simulink model "Circuito"  (R2014a)
settings: Solver=ode45  StartTime=0.0  StopTime=periodo  RelTol=1e-3
PreLoadFcn:
  | variables
InitFcn:
  | eval('variables');
  | variables
StartFcn:
  | variables
undefined symbols (not defined in the file): C, E, frecuencia, L, R, Rc, Rf, Rl, Rml
libraries: fl_lib x63, nesl_utility x4
settings Model: Creator=jhoan  LastModifiedBy=jhoan

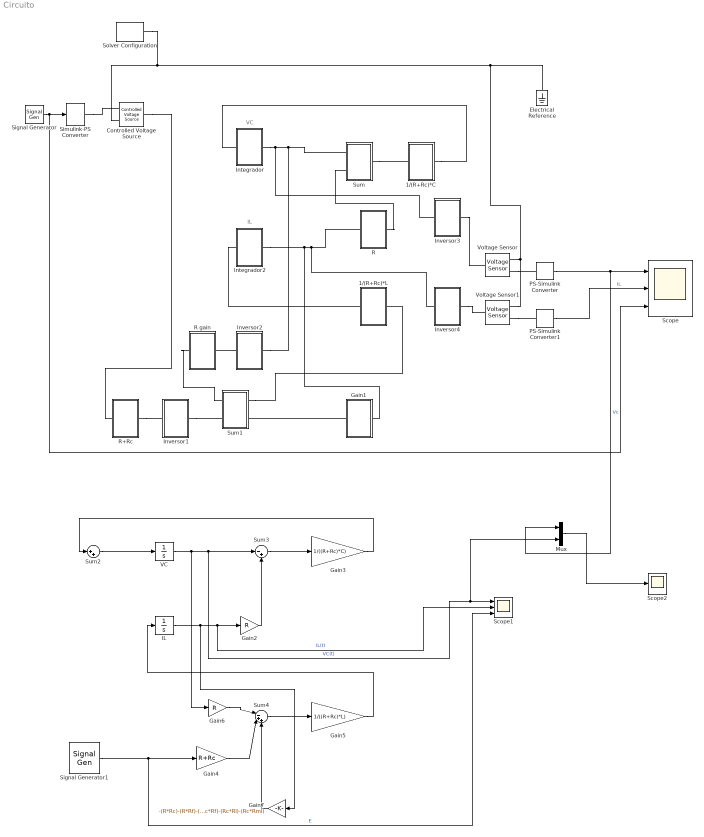
== system Circuito ==
  note: IL
  note: VC
  1/(R+Rc)*C : Subsystem
  1/(R+Rc)*L : Subsystem
  Controlled Voltage Source : fl_lib/Electrical/Electrical Sources/Controlled Voltage Source
  Electrical Reference : fl_lib/Electrical/Electrical Elements/Electrical Reference
  Gain1 : Subsystem
  Gain2 : Gain  Gain=R
  Gain3 : Gain  Gain=1/((R+Rc)*C)
  Gain4 : Gain  Gain=R+Rc
  Gain5 : Gain  Gain=1/((R+Rc)*L)
  Gain6 : Gain  Gain=R
  Gain7 : Gain  Gain=-(R*Rc)-(R*Rf)-(R*Rl)-(R*Rml)-(Rc*Rf)-(Rc*Rl)-(Rc*Rml)
  IL : Integrator
  Integrador : Subsystem
  Integrador2 : Subsystem
  Inversor1 : Subsystem
  Inversor2 : Subsystem
  Inversor3 : Subsystem
  Inversor4 : Subsystem
  Mux : Mux  Inputs=2
  PS-Simulink Converter : nesl_utility/PS-Simulink Converter  PhysicalDomain=network_engine_domain  SubClassName=ps_output  LeftPortType=input  RightPortType=output  PseudoPeriodic=off  Frequencies=[]  Unit=1  AffineConversion=off
  PS-Simulink Converter1 : nesl_utility/PS-Simulink Converter  PhysicalDomain=network_engine_domain  SubClassName=ps_output  LeftPortType=input  RightPortType=output  PseudoPeriodic=off  Frequencies=[]  Unit=1  AffineConversion=off
  R : Subsystem
  R gain : Subsystem
  R+Rc : Subsystem
  Scope : Scope  NumInputPorts=3
      settings: YMin=-5~-5~-5  YMax=5~5~5
  Scope1 : Scope  NumInputPorts=3
      settings: YMin=-5~-5~-5  YMax=5~5~5  SaveName=subSimulink
  Scope2 : Scope
      settings: SaveName=subSimulink1
  Signal Generator : SignalGenerator  WaveForm=square  Amplitude=E  Frequency=frecuencia
  Signal Generator1 : SignalGenerator  WaveForm=square  Amplitude=E  Frequency=frecuencia
  Simulink-PS Converter : nesl_utility/Simulink-PS Converter  PhysicalDomain=network_engine_domain  SubClassName=ps_input  LeftPortType=input  RightPortType=output  PseudoPeriodic=off  Frequencies=[]  NoiseDistribution=none  NoiseParameters=[]  Unit=1  AffineConversion=off  InputFiltering=off  SimscapeFilterOrder=1  InputFilterTimeConstant=0.001  UdotUserProvided=1
  Solver Configuration : nesl_utility/Solver Configuration  PhysicalDomain=network_engine_domain  SubClassName=solver  LeftPortType=input  RightPortType=generic  Accelerate=off  Tones=[]  Harmonics=[]  SimulateNoise=off  Profile=off  UseLocalSampling=off  EnableSwitchedLinearOptims=on  FrequencyDomain=off  UseCCode=off  RelTol=0.001  AbsTol=1e-06  MinStep=1e-09  ToWorkspace=off  DoDC=off  ResidualTolerance=1e-09  UseLocalSolver=off  LocalSolverChoice=NE_BACKWARD_EULER_ADVANCER  LocalSolverSampleTime=0.001  DoFixedCost=off  MaxNonlinIter=3  MaxModeIter=2  LinearAlgebra=Sparse  DelaysMemoryBudget=1024  AutomaticFiltering=on  FilteringTimeConstant=0.001
  Sum : Subsystem
  Sum1 : Subsystem
  Sum2 : Sum  Inputs=|++
  Sum3 : Sum  Inputs=|-+
  Sum4 : Sum  Inputs=|-++
  VC : Integrator
  Voltage Sensor : fl_lib/Electrical/Electrical Sensors/Voltage Sensor
  Voltage Sensor1 : fl_lib/Electrical/Electrical Sensors/Voltage Sensor
  wires:
  PS-Simulink Converter/1 -> Mux/1, Scope/1  "Vc"
  PS-Simulink Converter1/1 -> Scope/2  "IL"
  Signal Generator/1 -> Scope/3, Simulink-PS Converter/1
  Sum2/1 -> VC/1
  IL/1 -> Gain7/1, Scope1/2, Gain2/1  "IL(t)"
  VC/1 -> Gain6/1, Mux/2, Scope1/1, Sum3/1  "VC(t)"
  Gain2/1 -> Sum3/2
  Sum3/1 -> Gain3/1
  Gain3/1 -> Sum2/1
  Signal Generator1/1 -> Scope1/3, Gain4/1  "E"
  Gain4/1 -> Sum4/2
  Sum4/1 -> Gain5/1
  Gain6/1 -> Sum4/1
  Gain5/1 -> IL/1
  Gain7/1 -> Sum4/3
  Mux/1 -> Scope2/1
  connections:
  Solver Configuration/RConn1 -- Controlled Voltage Source/RConn2 -- Electrical Reference/LConn1 -- Voltage Sensor1/RConn2 -- Voltage Sensor/RConn2
  Integrador/RConn1 -- Inversor3/LConn1 -- Inversor2/LConn1 -- Sum/LConn1
  Integrador2/RConn1 -- Gain1/LConn1 -- Inversor4/LConn1 -- R/LConn1
  R/RConn1 -- Sum/LConn2
  Sum/RConn1 -- 1/(R+Rc)*C/LConn1
  1/(R+Rc)*C/RConn1 -- Integrador/LConn1
  Voltage Sensor/RConn1 -- PS-Simulink Converter/LConn1
  Simulink-PS Converter/RConn1 -- Controlled Voltage Source/RConn1
  Controlled Voltage Source/LConn1 -- R+Rc/LConn1
  Inversor2/RConn1 -- R gain/LConn1
  R gain/RConn1 -- Sum1/LConn1
  Sum1/RConn1 -- 1/(R+Rc)*L/LConn1
  1/(R+Rc)*L/RConn1 -- Integrador2/LConn1
  Voltage Sensor1/RConn1 -- PS-Simulink Converter1/LConn1
  R+Rc/RConn1 -- Inversor1/LConn1
  Inversor1/RConn1 -- Sum1/LConn2
  Gain1/RConn1 -- Sum1/RConn2
  Inversor3/RConn1 -- Voltage Sensor/LConn1
  Inversor4/RConn1 -- Voltage Sensor1/LConn1

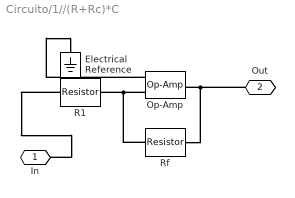
== system Circuito/1//(R+Rc)*C ==
  Electrical Reference : fl_lib/Electrical/Electrical Elements/Electrical Reference
  Op-Amp : fl_lib/Electrical/Electrical Elements/Op-Amp  outI_specify=off  outI_priority=High  outI=0 A
  R1 : fl_lib/Electrical/Electrical Elements/Resistor  R=(R+Rc)*C Ohm  i_specify=off  i_priority=High  i=0 A  v_specify=off  v_priority=High  v=0 V
  Rf : fl_lib/Electrical/Electrical Elements/Resistor  R=1 Ohm  i_specify=off  i_priority=High  i=0 A  v_specify=off  v_priority=High  v=0 V
  In : PMIOPort  Port=1  Side=Left
  Out : PMIOPort  Port=2  Side=Right
  connections:
  R1/LConn1 -- In/RConn1
  Out/RConn1 -- Rf/RConn1 -- Op-Amp/RConn1
  Op-Amp/LConn1 -- Electrical Reference/LConn1
  Op-Amp/LConn2 -- Rf/LConn1 -- R1/RConn1

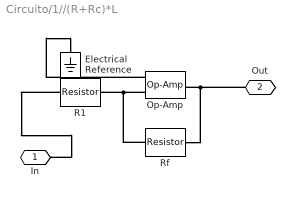
== system Circuito/1//(R+Rc)*L ==
  Electrical Reference : fl_lib/Electrical/Electrical Elements/Electrical Reference
  Op-Amp : fl_lib/Electrical/Electrical Elements/Op-Amp  outI_specify=off  outI_priority=High  outI=0 A
  R1 : fl_lib/Electrical/Electrical Elements/Resistor  R=(R+Rc)*L Ohm  i_specify=off  i_priority=High  i=0 A  v_specify=off  v_priority=High  v=0 V
  Rf : fl_lib/Electrical/Electrical Elements/Resistor  R=1 Ohm  i_specify=off  i_priority=High  i=0 A  v_specify=off  v_priority=High  v=0 V
  In : PMIOPort  Port=1  Side=Left
  Out : PMIOPort  Port=2  Side=Right
  connections:
  R1/LConn1 -- In/RConn1
  Out/RConn1 -- Rf/RConn1 -- Op-Amp/RConn1
  Op-Amp/LConn1 -- Electrical Reference/LConn1
  Op-Amp/LConn2 -- Rf/LConn1 -- R1/RConn1

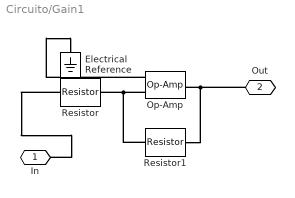
== system Circuito/Gain1 ==
  Electrical Reference : fl_lib/Electrical/Electrical Elements/Electrical Reference
  Op-Amp : fl_lib/Electrical/Electrical Elements/Op-Amp  outI_specify=off  outI_priority=High  outI=0 A
  Resistor : fl_lib/Electrical/Electrical Elements/Resistor  R=1 Ohm  i_specify=off  i_priority=High  i=0 A  v_specify=off  v_priority=High  v=0 V
  Resistor1 : fl_lib/Electrical/Electrical Elements/Resistor  R=(R*Rc)+(R*Rf)+(R*Rl)+(R*Rml)+(Rc*Rf)+(Rc*Rl)+(Rc*Rml) Ohm  i_specify=off  i_priority=High  i=0 A  v_specify=off  v_priority=High  v=0 V
  In : PMIOPort  Port=1  Side=Left
  Out : PMIOPort  Port=2  Side=Right
  connections:
  Resistor/LConn1 -- In/RConn1
  Out/RConn1 -- Resistor1/RConn1 -- Op-Amp/RConn1
  Op-Amp/LConn1 -- Electrical Reference/LConn1
  Op-Amp/LConn2 -- Resistor1/LConn1 -- Resistor/RConn1

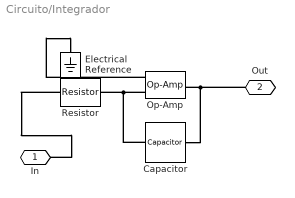
== system Circuito/Integrador ==
  Capacitor : fl_lib/Electrical/Electrical Elements/Capacitor  c=1e-6 F  r=1e-6 Ohm  g=0 1/Ohm  i_specify=off  i_priority=High  i=0 A  v_specify=off  v_priority=High  v=0 V  vc_specify=off  vc_priority=High  vc=0 V
  Electrical Reference : fl_lib/Electrical/Electrical Elements/Electrical Reference
  Op-Amp : fl_lib/Electrical/Electrical Elements/Op-Amp  outI_specify=off  outI_priority=High  outI=0 A
  Resistor : fl_lib/Electrical/Electrical Elements/Resistor  R=1 MOhm  i_specify=off  i_priority=High  i=0 A  v_specify=off  v_priority=High  v=0 V
  In : PMIOPort  Port=1  Side=Left
  Out : PMIOPort  Port=2  Side=Right
  connections:
  Resistor/LConn1 -- In/RConn1
  Capacitor/RConn1 -- Out/RConn1 -- Op-Amp/RConn1
  Op-Amp/LConn1 -- Electrical Reference/LConn1
  Op-Amp/LConn2 -- Capacitor/LConn1 -- Resistor/RConn1

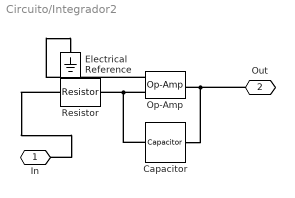
== system Circuito/Integrador2 ==
  Capacitor : fl_lib/Electrical/Electrical Elements/Capacitor  c=1e-6 F  r=1e-6 Ohm  g=0 1/Ohm  i_specify=off  i_priority=High  i=0 A  v_specify=off  v_priority=High  v=0 V  vc_specify=off  vc_priority=High  vc=0 V
  Electrical Reference : fl_lib/Electrical/Electrical Elements/Electrical Reference
  Op-Amp : fl_lib/Electrical/Electrical Elements/Op-Amp  outI_specify=off  outI_priority=High  outI=0 A
  Resistor : fl_lib/Electrical/Electrical Elements/Resistor  R=1 MOhm  i_specify=off  i_priority=High  i=0 A  v_specify=off  v_priority=High  v=0 V
  In : PMIOPort  Port=1  Side=Left
  Out : PMIOPort  Port=2  Side=Right
  connections:
  Resistor/LConn1 -- In/RConn1
  Capacitor/RConn1 -- Out/RConn1 -- Op-Amp/RConn1
  Op-Amp/LConn1 -- Electrical Reference/LConn1
  Op-Amp/LConn2 -- Capacitor/LConn1 -- Resistor/RConn1

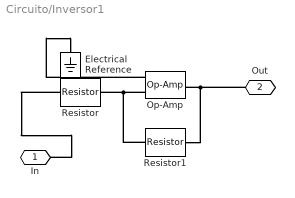
== system Circuito/Inversor1 ==
  Electrical Reference : fl_lib/Electrical/Electrical Elements/Electrical Reference
  Op-Amp : fl_lib/Electrical/Electrical Elements/Op-Amp  outI_specify=off  outI_priority=High  outI=0 A
  Resistor : fl_lib/Electrical/Electrical Elements/Resistor  R=1 kOhm  i_specify=off  i_priority=High  i=0 A  v_specify=off  v_priority=High  v=0 V
  Resistor1 : fl_lib/Electrical/Electrical Elements/Resistor  R=1 kOhm  i_specify=off  i_priority=High  i=0 A  v_specify=off  v_priority=High  v=0 V
  In : PMIOPort  Port=1  Side=Left
  Out : PMIOPort  Port=2  Side=Right
  connections:
  Resistor/LConn1 -- In/RConn1
  Out/RConn1 -- Resistor1/RConn1 -- Op-Amp/RConn1
  Op-Amp/LConn1 -- Electrical Reference/LConn1
  Op-Amp/LConn2 -- Resistor1/LConn1 -- Resistor/RConn1

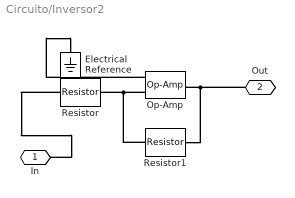
== system Circuito/Inversor2 ==
  Electrical Reference : fl_lib/Electrical/Electrical Elements/Electrical Reference
  Op-Amp : fl_lib/Electrical/Electrical Elements/Op-Amp  outI_specify=off  outI_priority=High  outI=0 A
  Resistor : fl_lib/Electrical/Electrical Elements/Resistor  R=1 kOhm  i_specify=off  i_priority=High  i=0 A  v_specify=off  v_priority=High  v=0 V
  Resistor1 : fl_lib/Electrical/Electrical Elements/Resistor  R=1 kOhm  i_specify=off  i_priority=High  i=0 A  v_specify=off  v_priority=High  v=0 V
  In : PMIOPort  Port=1  Side=Left
  Out : PMIOPort  Port=2  Side=Right
  connections:
  Resistor/LConn1 -- In/RConn1
  Out/RConn1 -- Resistor1/RConn1 -- Op-Amp/RConn1
  Op-Amp/LConn1 -- Electrical Reference/LConn1
  Op-Amp/LConn2 -- Resistor1/LConn1 -- Resistor/RConn1

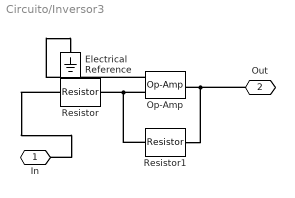
== system Circuito/Inversor3 ==
  Electrical Reference : fl_lib/Electrical/Electrical Elements/Electrical Reference
  Op-Amp : fl_lib/Electrical/Electrical Elements/Op-Amp  outI_specify=off  outI_priority=High  outI=0 A
  Resistor : fl_lib/Electrical/Electrical Elements/Resistor  R=1 kOhm  i_specify=off  i_priority=High  i=0 A  v_specify=off  v_priority=High  v=0 V
  Resistor1 : fl_lib/Electrical/Electrical Elements/Resistor  R=1 kOhm  i_specify=off  i_priority=High  i=0 A  v_specify=off  v_priority=High  v=0 V
  In : PMIOPort  Port=1  Side=Left
  Out : PMIOPort  Port=2  Side=Right
  connections:
  Resistor/LConn1 -- In/RConn1
  Out/RConn1 -- Resistor1/RConn1 -- Op-Amp/RConn1
  Op-Amp/LConn1 -- Electrical Reference/LConn1
  Op-Amp/LConn2 -- Resistor1/LConn1 -- Resistor/RConn1

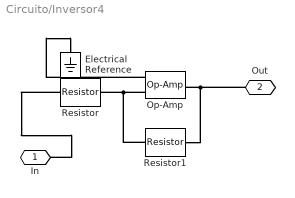
== system Circuito/Inversor4 ==
  Electrical Reference : fl_lib/Electrical/Electrical Elements/Electrical Reference
  Op-Amp : fl_lib/Electrical/Electrical Elements/Op-Amp  outI_specify=off  outI_priority=High  outI=0 A
  Resistor : fl_lib/Electrical/Electrical Elements/Resistor  R=1 kOhm  i_specify=off  i_priority=High  i=0 A  v_specify=off  v_priority=High  v=0 V
  Resistor1 : fl_lib/Electrical/Electrical Elements/Resistor  R=1 kOhm  i_specify=off  i_priority=High  i=0 A  v_specify=off  v_priority=High  v=0 V
  In : PMIOPort  Port=1  Side=Left
  Out : PMIOPort  Port=2  Side=Right
  connections:
  Resistor/LConn1 -- In/RConn1
  Out/RConn1 -- Resistor1/RConn1 -- Op-Amp/RConn1
  Op-Amp/LConn1 -- Electrical Reference/LConn1
  Op-Amp/LConn2 -- Resistor1/LConn1 -- Resistor/RConn1

== system Circuito/R ==
  Electrical Reference : fl_lib/Electrical/Electrical Elements/Electrical Reference
  Op-Amp : fl_lib/Electrical/Electrical Elements/Op-Amp  outI_specify=off  outI_priority=High  outI=0 A
  R1 : fl_lib/Electrical/Electrical Elements/Resistor  R=1 Ohm  i_specify=off  i_priority=High  i=0 A  v_specify=off  v_priority=High  v=0 V
  Rf : fl_lib/Electrical/Electrical Elements/Resistor  R=R Ohm  i_specify=off  i_priority=High  i=0 A  v_specify=off  v_priority=High  v=0 V
  In : PMIOPort  Port=1  Side=Left
  Out : PMIOPort  Port=2  Side=Right
  connections:
  R1/LConn1 -- In/RConn1
  Out/RConn1 -- Rf/RConn1 -- Op-Amp/RConn1
  Op-Amp/LConn1 -- Electrical Reference/LConn1
  Op-Amp/LConn2 -- Rf/LConn1 -- R1/RConn1

== system Circuito/R gain ==
  Electrical Reference : fl_lib/Electrical/Electrical Elements/Electrical Reference
  Op-Amp : fl_lib/Electrical/Electrical Elements/Op-Amp  outI_specify=off  outI_priority=High  outI=0 A
  Resistor : fl_lib/Electrical/Electrical Elements/Resistor  R=1 Ohm  i_specify=off  i_priority=High  i=0 A  v_specify=off  v_priority=High  v=0 V
  Resistor1 : fl_lib/Electrical/Electrical Elements/Resistor  R=R Ohm  i_specify=off  i_priority=High  i=0 A  v_specify=off  v_priority=High  v=0 V
  In : PMIOPort  Port=1  Side=Left
  Out : PMIOPort  Port=2  Side=Right
  connections:
  Resistor/LConn1 -- In/RConn1
  Out/RConn1 -- Resistor1/RConn1 -- Op-Amp/RConn1
  Op-Amp/LConn1 -- Electrical Reference/LConn1
  Op-Amp/LConn2 -- Resistor1/LConn1 -- Resistor/RConn1

== system Circuito/R+Rc ==
  Electrical Reference : fl_lib/Electrical/Electrical Elements/Electrical Reference
  Op-Amp : fl_lib/Electrical/Electrical Elements/Op-Amp  outI_specify=off  outI_priority=High  outI=0 A
  R1 : fl_lib/Electrical/Electrical Elements/Resistor  R=1 Ohm  i_specify=off  i_priority=High  i=0 A  v_specify=off  v_priority=High  v=0 V
  Rf : fl_lib/Electrical/Electrical Elements/Resistor  R=R+Rc Ohm  i_specify=off  i_priority=High  i=0 A  v_specify=off  v_priority=High  v=0 V
  In : PMIOPort  Port=1  Side=Left
  Out : PMIOPort  Port=2  Side=Right
  connections:
  R1/LConn1 -- In/RConn1
  Out/RConn1 -- Rf/RConn1 -- Op-Amp/RConn1
  Op-Amp/LConn1 -- Electrical Reference/LConn1
  Op-Amp/LConn2 -- Rf/LConn1 -- R1/RConn1

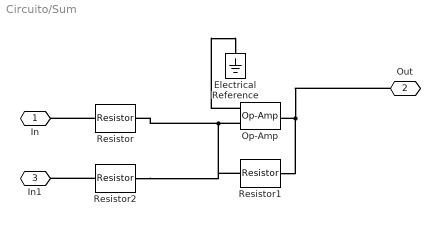
== system Circuito/Sum ==
  Electrical Reference : fl_lib/Electrical/Electrical Elements/Electrical Reference
  Op-Amp : fl_lib/Electrical/Electrical Elements/Op-Amp  outI_specify=off  outI_priority=High  outI=0 A
  Resistor : fl_lib/Electrical/Electrical Elements/Resistor  R=1 kOhm  i_specify=off  i_priority=High  i=0 A  v_specify=off  v_priority=High  v=0 V
  Resistor1 : fl_lib/Electrical/Electrical Elements/Resistor  R=1 kOhm  i_specify=off  i_priority=High  i=0 A  v_specify=off  v_priority=High  v=0 V
  Resistor2 : fl_lib/Electrical/Electrical Elements/Resistor  R=1 kOhm  i_specify=off  i_priority=High  i=0 A  v_specify=off  v_priority=High  v=0 V
  In : PMIOPort  Port=1  Side=Left
  Out : PMIOPort  Port=2  Side=Right
  In1 : PMIOPort  Port=3  Side=Left
  connections:
  Resistor/LConn1 -- In/RConn1
  Out/RConn1 -- Resistor1/RConn1 -- Op-Amp/RConn1
  Op-Amp/LConn1 -- Electrical Reference/LConn1
  Op-Amp/LConn2 -- Resistor2/RConn1 -- Resistor1/LConn1 -- Resistor/RConn1
  Resistor2/LConn1 -- In1/RConn1

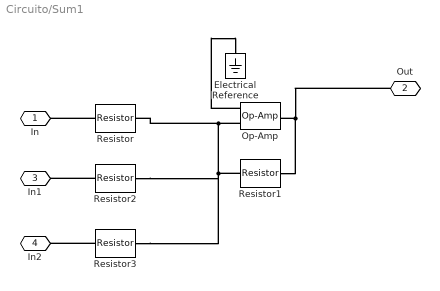
== system Circuito/Sum1 ==
  Electrical Reference : fl_lib/Electrical/Electrical Elements/Electrical Reference
  Op-Amp : fl_lib/Electrical/Electrical Elements/Op-Amp  outI_specify=off  outI_priority=High  outI=0 A
  Resistor{,1..3} (4 alike) : fl_lib/Electrical/Electrical Elements/Resistor  R=1 kOhm  i_specify=off  i_priority=High  i=0 A  v_specify=off  v_priority=High  v=0 V
  In : PMIOPort  Port=1  Side=Left
  Out : PMIOPort  Port=2  Side=Right
  In1 : PMIOPort  Port=3  Side=Left
  In2 : PMIOPort  Port=4  Side=Right
  connections:
  Resistor/LConn1 -- In/RConn1
  Out/RConn1 -- Op-Amp/RConn1 -- Resistor1/RConn1
  Op-Amp/LConn1 -- Electrical Reference/LConn1
  Op-Amp/LConn2 -- Resistor/RConn1 -- Resistor3/RConn1 -- Resistor2/RConn1 -- Resistor1/LConn1
  Resistor2/LConn1 -- In1/RConn1
  Resistor3/LConn1 -- In2/RConn1
